simulink model "AFDNFSmodelMPA"  (Simulink 8.8)
settings: Solver=ode45  StartTime=0.0  StopTime=100  FixedStep=1e-3  RelTol=1e-6  EnableMultiTasking=on
InitFcn:
  | run('Methods/AFDSimInit')
  | load('SampleDatcomData.mat')
values from neighbouring files (symbols this model uses):
  nfs = TransferFunction('Plot','true')    [Main.m]    (also in NFSDatabase.sldd = SI
                Imperial
                28184.4409185639)
undefined symbols (not defined in the file or in its folder): datcom, desired, K_lat, K_long, Kobsvlat, Kobsvlong, lat, latsys, long, longsys, Newton, Raphson, sigbuilder_block
libraries: aerolibutil x13, aerolibtransform2 x1, aerolibasang x1
(part 3 of 3)

== system AFDNFSmodelMPA/Nonlinear Flight Simulator/Forces&Moments/Digital DATCOM v1.0.2/Deflection/Aerodynamic Forces and Moments/CG-CP Transformation/Body2Stability ==
  alpha : Inport
  Constant{,1,3..4} (4 alike) : Constant  Value=0
  Constant2 : Constant
  Create 3x3 Matrix : aerolibutil/Create 3x3 Matrix
  Trigonometric Function2 : Trigonometry  Operator=sincos
  Unary Minus : UnaryMinus
  Ts/b : Outport
  wires:
  alpha/1 -> Trigonometric Function2/1
  Trigonometric Function2/2 -> Create 3x3 Matrix/9, Create 3x3 Matrix/1
  Constant4/1 -> Create 3x3 Matrix/8
  Unary Minus/1 -> Create 3x3 Matrix/7
  Trigonometric Function2/1 -> Unary Minus/1, Create 3x3 Matrix/3
  Constant3/1 -> Create 3x3 Matrix/6
  Constant2/1 -> Create 3x3 Matrix/5
  Constant1/1 -> Create 3x3 Matrix/4
  Constant/1 -> Create 3x3 Matrix/2
  Create 3x3 Matrix/1 -> Ts/b/1

== system AFDNFSmodelMPA/Nonlinear Flight Simulator/Forces&Moments/Digital DATCOM v1.0.2/Deflection/Aerodynamic Forces and Moments/CG-CP Transformation/Incidence, Sideslip, & Airspeed ==
  Vb : Inport  Unit=m/s
  Airspeed : Sqrt  AlgorithmType=Newton-Raphson  SaturateOnIntegerOverflow=on
  Dot Product : DotProduct  InputSameDT=on  OutDataTypeStr=Inherit: Inherit via internal rule
  Incidence : Trigonometry  Operator=atan2
  Product : Product  Inputs=*/  SaturateOnIntegerOverflow=on  OutDataTypeStr=Inherit: Same as first input
  Selector : Selector  InputPortWidth=3  IndexOptions=Index vector (dialog)  Indices=[2]  OutputSizes=1
  Selector1 : Selector  InputPortWidth=3  IndexOptions=Index vector (dialog)  Indices=[3]  OutputSizes=1
  Selector2 : Selector  InputPortWidth=3  IndexOptions=Index vector (dialog)  Indices=[1]  OutputSizes=1
  Sideslip : Trigonometry  Operator=asin
  Alpha : Outport  Unit=rad  InitialOutput=0
  Beta : Outport  Port=2  Unit=rad  InitialOutput=0
  V : Outport  Port=3  Unit=m/s  InitialOutput=0
  wires:
  Selector/1 -> Product/1
  Sideslip/1 -> Beta/1
  Vb/1 -> Dot Product/2, Dot Product/1, Selector/1, Selector2/1, Selector1/1
  Incidence/1 -> Alpha/1
  Airspeed/1 -> V/1, Product/2
  Dot Product/1 -> Airspeed/1
  Selector2/1 -> Incidence/2
  Selector1/1 -> Incidence/1
  Product/1 -> Sideslip/1

== system AFDNFSmodelMPA/Nonlinear Flight Simulator/Forces&Moments/Digital DATCOM v1.0.2/Deflection/Aerodynamic Forces and Moments/Force Transformation/Body2Stability ==
  alpha : Inport
  Constant{,1,3..4} (4 alike) : Constant  Value=0
  Constant2 : Constant
  Create 3x3 Matrix : aerolibutil/Create 3x3 Matrix
  Trigonometric Function2 : Trigonometry  Operator=sincos
  Unary Minus : UnaryMinus
  Ts/b : Outport
  wires:
  alpha/1 -> Trigonometric Function2/1
  Trigonometric Function2/2 -> Create 3x3 Matrix/9, Create 3x3 Matrix/1
  Constant4/1 -> Create 3x3 Matrix/8
  Unary Minus/1 -> Create 3x3 Matrix/7
  Trigonometric Function2/1 -> Unary Minus/1, Create 3x3 Matrix/3
  Constant3/1 -> Create 3x3 Matrix/6
  Constant2/1 -> Create 3x3 Matrix/5
  Constant1/1 -> Create 3x3 Matrix/4
  Constant/1 -> Create 3x3 Matrix/2
  Create 3x3 Matrix/1 -> Ts/b/1

== system AFDNFSmodelMPA/Nonlinear Flight Simulator/Forces&Moments/Digital DATCOM v1.0.2/Deflection/Aerodynamic Forces and Moments/Force Transformation/Incidence, Sideslip, & Airspeed ==
  Vb : Inport  Unit=m/s
  Airspeed : Sqrt  AlgorithmType=Newton-Raphson  SaturateOnIntegerOverflow=on
  Dot Product : DotProduct  InputSameDT=on  OutDataTypeStr=Inherit: Inherit via internal rule
  Incidence : Trigonometry  Operator=atan2
  Product : Product  Inputs=*/  SaturateOnIntegerOverflow=on  OutDataTypeStr=Inherit: Same as first input
  Selector : Selector  InputPortWidth=3  IndexOptions=Index vector (dialog)  Indices=[2]  OutputSizes=1
  Selector1 : Selector  InputPortWidth=3  IndexOptions=Index vector (dialog)  Indices=[3]  OutputSizes=1
  Selector2 : Selector  InputPortWidth=3  IndexOptions=Index vector (dialog)  Indices=[1]  OutputSizes=1
  Sideslip : Trigonometry  Operator=asin
  Alpha : Outport  Unit=rad  InitialOutput=0
  Beta : Outport  Port=2  Unit=rad  InitialOutput=0
  V : Outport  Port=3  Unit=m/s  InitialOutput=0
  wires:
  Selector/1 -> Product/1
  Sideslip/1 -> Beta/1
  Vb/1 -> Dot Product/2, Dot Product/1, Selector/1, Selector2/1, Selector1/1
  Incidence/1 -> Alpha/1
  Airspeed/1 -> V/1, Product/2
  Dot Product/1 -> Airspeed/1
  Selector2/1 -> Incidence/2
  Selector1/1 -> Incidence/1
  Product/1 -> Sideslip/1

== system AFDNFSmodelMPA/Nonlinear Flight Simulator/Forces&Moments/Digital DATCOM v1.0.2/Deflection/Aerodynamic Forces and Moments/Moment Transformation/Body2Stability ==
  alpha : Inport
  Constant{,1,3..4} (4 alike) : Constant  Value=0
  Constant2 : Constant
  Create 3x3 Matrix : aerolibutil/Create 3x3 Matrix
  Trigonometric Function2 : Trigonometry  Operator=sincos
  Unary Minus : UnaryMinus
  Ts/b : Outport
  wires:
  Create 3x3 Matrix/1 -> Ts/b/1
  Constant/1 -> Create 3x3 Matrix/2
  Constant1/1 -> Create 3x3 Matrix/4
  Constant2/1 -> Create 3x3 Matrix/5
  Constant3/1 -> Create 3x3 Matrix/6
  Trigonometric Function2/1 -> Create 3x3 Matrix/3, Unary Minus/1
  Unary Minus/1 -> Create 3x3 Matrix/7
  Constant4/1 -> Create 3x3 Matrix/8
  Trigonometric Function2/2 -> Create 3x3 Matrix/1, Create 3x3 Matrix/9
  alpha/1 -> Trigonometric Function2/1

== system AFDNFSmodelMPA/Nonlinear Flight Simulator/Forces&Moments/Digital DATCOM v1.0.2/Deflection/Aerodynamic Forces and Moments/Moment Transformation/Incidence, Sideslip, & Airspeed ==
  Vb : Inport  Unit=m/s
  Airspeed : Sqrt  AlgorithmType=Newton-Raphson  SaturateOnIntegerOverflow=on
  Dot Product : DotProduct  InputSameDT=on  OutDataTypeStr=Inherit: Inherit via internal rule
  Incidence : Trigonometry  Operator=atan2
  Product : Product  Inputs=*/  SaturateOnIntegerOverflow=on  OutDataTypeStr=Inherit: Same as first input
  Selector : Selector  InputPortWidth=3  IndexOptions=Index vector (dialog)  Indices=[2]  OutputSizes=1
  Selector1 : Selector  InputPortWidth=3  IndexOptions=Index vector (dialog)  Indices=[3]  OutputSizes=1
  Selector2 : Selector  InputPortWidth=3  IndexOptions=Index vector (dialog)  Indices=[1]  OutputSizes=1
  Sideslip : Trigonometry  Operator=asin
  Alpha : Outport  Unit=rad  InitialOutput=0
  Beta : Outport  Port=2  Unit=rad  InitialOutput=0
  V : Outport  Port=3  Unit=m/s  InitialOutput=0
  wires:
  Product/1 -> Sideslip/1
  Selector1/1 -> Incidence/1
  Selector2/1 -> Incidence/2
  Dot Product/1 -> Airspeed/1
  Airspeed/1 -> Product/2, V/1
  Incidence/1 -> Alpha/1
  Vb/1 -> Selector1/1, Selector2/1, Selector/1, Dot Product/1, Dot Product/2
  Sideslip/1 -> Beta/1
  Selector/1 -> Product/1

== system AFDNFSmodelMPA/Nonlinear Flight Simulator/Forces&Moments/Digital DATCOM v1.0.2/Dynamic Contribution/Aerodynamic Forces and Moments Stability Axis/CG-CP Transformation/Body2Stability ==
  alpha : Inport
  Constant{,1,3..4} (4 alike) : Constant  Value=0
  Constant2 : Constant
  Create 3x3 Matrix : aerolibutil/Create 3x3 Matrix
  Trigonometric Function2 : Trigonometry  Operator=sincos
  Unary Minus : UnaryMinus
  Ts/b : Outport
  wires:
  alpha/1 -> Trigonometric Function2/1
  Trigonometric Function2/2 -> Create 3x3 Matrix/9, Create 3x3 Matrix/1
  Constant4/1 -> Create 3x3 Matrix/8
  Unary Minus/1 -> Create 3x3 Matrix/7
  Trigonometric Function2/1 -> Unary Minus/1, Create 3x3 Matrix/3
  Constant3/1 -> Create 3x3 Matrix/6
  Constant2/1 -> Create 3x3 Matrix/5
  Constant1/1 -> Create 3x3 Matrix/4
  Constant/1 -> Create 3x3 Matrix/2
  Create 3x3 Matrix/1 -> Ts/b/1

== system AFDNFSmodelMPA/Nonlinear Flight Simulator/Forces&Moments/Digital DATCOM v1.0.2/Dynamic Contribution/Aerodynamic Forces and Moments Stability Axis/CG-CP Transformation/Incidence, Sideslip, & Airspeed ==
  Vb : Inport  Unit=m/s
  Airspeed : Sqrt  AlgorithmType=Newton-Raphson  SaturateOnIntegerOverflow=on
  Dot Product : DotProduct  InputSameDT=on  OutDataTypeStr=Inherit: Inherit via internal rule
  Incidence : Trigonometry  Operator=atan2
  Product : Product  Inputs=*/  SaturateOnIntegerOverflow=on  OutDataTypeStr=Inherit: Same as first input
  Selector : Selector  InputPortWidth=3  IndexOptions=Index vector (dialog)  Indices=[2]  OutputSizes=1
  Selector1 : Selector  InputPortWidth=3  IndexOptions=Index vector (dialog)  Indices=[3]  OutputSizes=1
  Selector2 : Selector  InputPortWidth=3  IndexOptions=Index vector (dialog)  Indices=[1]  OutputSizes=1
  Sideslip : Trigonometry  Operator=asin
  Alpha : Outport  Unit=rad  InitialOutput=0
  Beta : Outport  Port=2  Unit=rad  InitialOutput=0
  V : Outport  Port=3  Unit=m/s  InitialOutput=0
  wires:
  Selector/1 -> Product/1
  Sideslip/1 -> Beta/1
  Vb/1 -> Dot Product/2, Dot Product/1, Selector/1, Selector2/1, Selector1/1
  Incidence/1 -> Alpha/1
  Airspeed/1 -> V/1, Product/2
  Dot Product/1 -> Airspeed/1
  Selector2/1 -> Incidence/2
  Selector1/1 -> Incidence/1
  Product/1 -> Sideslip/1

== system AFDNFSmodelMPA/Nonlinear Flight Simulator/Forces&Moments/Digital DATCOM v1.0.2/Dynamic Contribution/Aerodynamic Forces and Moments Stability Axis/Force Transformation/Body2Stability ==
  alpha : Inport
  Constant{,1,3..4} (4 alike) : Constant  Value=0
  Constant2 : Constant
  Create 3x3 Matrix : aerolibutil/Create 3x3 Matrix
  Trigonometric Function2 : Trigonometry  Operator=sincos
  Unary Minus : UnaryMinus
  Ts/b : Outport
  wires:
  alpha/1 -> Trigonometric Function2/1
  Trigonometric Function2/2 -> Create 3x3 Matrix/9, Create 3x3 Matrix/1
  Constant4/1 -> Create 3x3 Matrix/8
  Unary Minus/1 -> Create 3x3 Matrix/7
  Trigonometric Function2/1 -> Unary Minus/1, Create 3x3 Matrix/3
  Constant3/1 -> Create 3x3 Matrix/6
  Constant2/1 -> Create 3x3 Matrix/5
  Constant1/1 -> Create 3x3 Matrix/4
  Constant/1 -> Create 3x3 Matrix/2
  Create 3x3 Matrix/1 -> Ts/b/1

== system AFDNFSmodelMPA/Nonlinear Flight Simulator/Forces&Moments/Digital DATCOM v1.0.2/Dynamic Contribution/Aerodynamic Forces and Moments Stability Axis/Force Transformation/Incidence, Sideslip, & Airspeed ==
  Vb : Inport  Unit=m/s
  Airspeed : Sqrt  AlgorithmType=Newton-Raphson  SaturateOnIntegerOverflow=on
  Dot Product : DotProduct  InputSameDT=on  OutDataTypeStr=Inherit: Inherit via internal rule
  Incidence : Trigonometry  Operator=atan2
  Product : Product  Inputs=*/  SaturateOnIntegerOverflow=on  OutDataTypeStr=Inherit: Same as first input
  Selector : Selector  InputPortWidth=3  IndexOptions=Index vector (dialog)  Indices=[2]  OutputSizes=1
  Selector1 : Selector  InputPortWidth=3  IndexOptions=Index vector (dialog)  Indices=[3]  OutputSizes=1
  Selector2 : Selector  InputPortWidth=3  IndexOptions=Index vector (dialog)  Indices=[1]  OutputSizes=1
  Sideslip : Trigonometry  Operator=asin
  Alpha : Outport  Unit=rad  InitialOutput=0
  Beta : Outport  Port=2  Unit=rad  InitialOutput=0
  V : Outport  Port=3  Unit=m/s  InitialOutput=0
  wires:
  Selector/1 -> Product/1
  Sideslip/1 -> Beta/1
  Vb/1 -> Dot Product/2, Dot Product/1, Selector/1, Selector2/1, Selector1/1
  Incidence/1 -> Alpha/1
  Airspeed/1 -> V/1, Product/2
  Dot Product/1 -> Airspeed/1
  Selector2/1 -> Incidence/2
  Selector1/1 -> Incidence/1
  Product/1 -> Sideslip/1

== system AFDNFSmodelMPA/Nonlinear Flight Simulator/Forces&Moments/Digital DATCOM v1.0.2/Dynamic Contribution/Aerodynamic Forces and Moments Stability Axis/Moment Transformation/Body2Stability ==
  alpha : Inport
  Constant{,1,3..4} (4 alike) : Constant  Value=0
  Constant2 : Constant
  Create 3x3 Matrix : aerolibutil/Create 3x3 Matrix
  Trigonometric Function2 : Trigonometry  Operator=sincos
  Unary Minus : UnaryMinus
  Ts/b : Outport
  wires:
  Create 3x3 Matrix/1 -> Ts/b/1
  Constant/1 -> Create 3x3 Matrix/2
  Constant1/1 -> Create 3x3 Matrix/4
  Constant2/1 -> Create 3x3 Matrix/5
  Constant3/1 -> Create 3x3 Matrix/6
  Trigonometric Function2/1 -> Create 3x3 Matrix/3, Unary Minus/1
  Unary Minus/1 -> Create 3x3 Matrix/7
  Constant4/1 -> Create 3x3 Matrix/8
  Trigonometric Function2/2 -> Create 3x3 Matrix/1, Create 3x3 Matrix/9
  alpha/1 -> Trigonometric Function2/1

== system AFDNFSmodelMPA/Nonlinear Flight Simulator/Forces&Moments/Digital DATCOM v1.0.2/Dynamic Contribution/Aerodynamic Forces and Moments Stability Axis/Moment Transformation/Incidence, Sideslip, & Airspeed ==
  Vb : Inport  Unit=m/s
  Airspeed : Sqrt  AlgorithmType=Newton-Raphson  SaturateOnIntegerOverflow=on
  Dot Product : DotProduct  InputSameDT=on  OutDataTypeStr=Inherit: Inherit via internal rule
  Incidence : Trigonometry  Operator=atan2
  Product : Product  Inputs=*/  SaturateOnIntegerOverflow=on  OutDataTypeStr=Inherit: Same as first input
  Selector : Selector  InputPortWidth=3  IndexOptions=Index vector (dialog)  Indices=[2]  OutputSizes=1
  Selector1 : Selector  InputPortWidth=3  IndexOptions=Index vector (dialog)  Indices=[3]  OutputSizes=1
  Selector2 : Selector  InputPortWidth=3  IndexOptions=Index vector (dialog)  Indices=[1]  OutputSizes=1
  Sideslip : Trigonometry  Operator=asin
  Alpha : Outport  Unit=rad  InitialOutput=0
  Beta : Outport  Port=2  Unit=rad  InitialOutput=0
  V : Outport  Port=3  Unit=m/s  InitialOutput=0
  wires:
  Product/1 -> Sideslip/1
  Selector1/1 -> Incidence/1
  Selector2/1 -> Incidence/2
  Dot Product/1 -> Airspeed/1
  Airspeed/1 -> Product/2, V/1
  Incidence/1 -> Alpha/1
  Vb/1 -> Selector1/1, Selector2/1, Selector/1, Dot Product/1, Dot Product/2
  Sideslip/1 -> Beta/1
  Selector/1 -> Product/1

== system AFDNFSmodelMPA/Nonlinear Flight Simulator/Forces&Moments/Digital DATCOM v1.0.2/Static Contribution/Aerodynamic Forces and Moments/CG-CP Transformation/Body2Stability ==
  alpha : Inport
  Constant{,1,3..4} (4 alike) : Constant  Value=0
  Constant2 : Constant
  Create 3x3 Matrix : aerolibutil/Create 3x3 Matrix
  Trigonometric Function2 : Trigonometry  Operator=sincos
  Unary Minus : UnaryMinus
  Ts/b : Outport
  wires:
  alpha/1 -> Trigonometric Function2/1
  Trigonometric Function2/2 -> Create 3x3 Matrix/9, Create 3x3 Matrix/1
  Constant4/1 -> Create 3x3 Matrix/8
  Unary Minus/1 -> Create 3x3 Matrix/7
  Trigonometric Function2/1 -> Unary Minus/1, Create 3x3 Matrix/3
  Constant3/1 -> Create 3x3 Matrix/6
  Constant2/1 -> Create 3x3 Matrix/5
  Constant1/1 -> Create 3x3 Matrix/4
  Constant/1 -> Create 3x3 Matrix/2
  Create 3x3 Matrix/1 -> Ts/b/1

== system AFDNFSmodelMPA/Nonlinear Flight Simulator/Forces&Moments/Digital DATCOM v1.0.2/Static Contribution/Aerodynamic Forces and Moments/CG-CP Transformation/Incidence, Sideslip, & Airspeed ==
  Vb : Inport  Unit=m/s
  Airspeed : Sqrt  AlgorithmType=Newton-Raphson  SaturateOnIntegerOverflow=on
  Dot Product : DotProduct  InputSameDT=on  OutDataTypeStr=Inherit: Inherit via internal rule
  Incidence : Trigonometry  Operator=atan2
  Product : Product  Inputs=*/  SaturateOnIntegerOverflow=on  OutDataTypeStr=Inherit: Same as first input
  Selector : Selector  InputPortWidth=3  IndexOptions=Index vector (dialog)  Indices=[2]  OutputSizes=1
  Selector1 : Selector  InputPortWidth=3  IndexOptions=Index vector (dialog)  Indices=[3]  OutputSizes=1
  Selector2 : Selector  InputPortWidth=3  IndexOptions=Index vector (dialog)  Indices=[1]  OutputSizes=1
  Sideslip : Trigonometry  Operator=asin
  Alpha : Outport  Unit=rad  InitialOutput=0
  Beta : Outport  Port=2  Unit=rad  InitialOutput=0
  V : Outport  Port=3  Unit=m/s  InitialOutput=0
  wires:
  Selector/1 -> Product/1
  Sideslip/1 -> Beta/1
  Vb/1 -> Dot Product/2, Dot Product/1, Selector/1, Selector2/1, Selector1/1
  Incidence/1 -> Alpha/1
  Airspeed/1 -> V/1, Product/2
  Dot Product/1 -> Airspeed/1
  Selector2/1 -> Incidence/2
  Selector1/1 -> Incidence/1
  Product/1 -> Sideslip/1

== system AFDNFSmodelMPA/Nonlinear Flight Simulator/Forces&Moments/Digital DATCOM v1.0.2/Static Contribution/Aerodynamic Forces and Moments/Force Transformation/Body2Stability ==
  alpha : Inport
  Constant{,1,3..4} (4 alike) : Constant  Value=0
  Constant2 : Constant
  Create 3x3 Matrix : aerolibutil/Create 3x3 Matrix
  Trigonometric Function2 : Trigonometry  Operator=sincos
  Unary Minus : UnaryMinus
  Ts/b : Outport
  wires:
  alpha/1 -> Trigonometric Function2/1
  Trigonometric Function2/2 -> Create 3x3 Matrix/9, Create 3x3 Matrix/1
  Constant4/1 -> Create 3x3 Matrix/8
  Unary Minus/1 -> Create 3x3 Matrix/7
  Trigonometric Function2/1 -> Unary Minus/1, Create 3x3 Matrix/3
  Constant3/1 -> Create 3x3 Matrix/6
  Constant2/1 -> Create 3x3 Matrix/5
  Constant1/1 -> Create 3x3 Matrix/4
  Constant/1 -> Create 3x3 Matrix/2
  Create 3x3 Matrix/1 -> Ts/b/1

== system AFDNFSmodelMPA/Nonlinear Flight Simulator/Forces&Moments/Digital DATCOM v1.0.2/Static Contribution/Aerodynamic Forces and Moments/Force Transformation/Incidence, Sideslip, & Airspeed ==
  Vb : Inport  Unit=m/s
  Airspeed : Sqrt  AlgorithmType=Newton-Raphson  SaturateOnIntegerOverflow=on
  Dot Product : DotProduct  InputSameDT=on  OutDataTypeStr=Inherit: Inherit via internal rule
  Incidence : Trigonometry  Operator=atan2
  Product : Product  Inputs=*/  SaturateOnIntegerOverflow=on  OutDataTypeStr=Inherit: Same as first input
  Selector : Selector  InputPortWidth=3  IndexOptions=Index vector (dialog)  Indices=[2]  OutputSizes=1
  Selector1 : Selector  InputPortWidth=3  IndexOptions=Index vector (dialog)  Indices=[3]  OutputSizes=1
  Selector2 : Selector  InputPortWidth=3  IndexOptions=Index vector (dialog)  Indices=[1]  OutputSizes=1
  Sideslip : Trigonometry  Operator=asin
  Alpha : Outport  Unit=rad  InitialOutput=0
  Beta : Outport  Port=2  Unit=rad  InitialOutput=0
  V : Outport  Port=3  Unit=m/s  InitialOutput=0
  wires:
  Selector/1 -> Product/1
  Sideslip/1 -> Beta/1
  Vb/1 -> Dot Product/2, Dot Product/1, Selector/1, Selector2/1, Selector1/1
  Incidence/1 -> Alpha/1
  Airspeed/1 -> V/1, Product/2
  Dot Product/1 -> Airspeed/1
  Selector2/1 -> Incidence/2
  Selector1/1 -> Incidence/1
  Product/1 -> Sideslip/1

== system AFDNFSmodelMPA/Nonlinear Flight Simulator/Forces&Moments/Digital DATCOM v1.0.2/Static Contribution/Aerodynamic Forces and Moments/Moment Transformation/Body2Stability ==
  alpha : Inport
  Constant{,1,3..4} (4 alike) : Constant  Value=0
  Constant2 : Constant
  Create 3x3 Matrix : aerolibutil/Create 3x3 Matrix
  Trigonometric Function2 : Trigonometry  Operator=sincos
  Unary Minus : UnaryMinus
  Ts/b : Outport
  wires:
  Create 3x3 Matrix/1 -> Ts/b/1
  Constant/1 -> Create 3x3 Matrix/2
  Constant1/1 -> Create 3x3 Matrix/4
  Constant2/1 -> Create 3x3 Matrix/5
  Constant3/1 -> Create 3x3 Matrix/6
  Trigonometric Function2/1 -> Create 3x3 Matrix/3, Unary Minus/1
  Unary Minus/1 -> Create 3x3 Matrix/7
  Constant4/1 -> Create 3x3 Matrix/8
  Trigonometric Function2/2 -> Create 3x3 Matrix/1, Create 3x3 Matrix/9
  alpha/1 -> Trigonometric Function2/1

== system AFDNFSmodelMPA/Nonlinear Flight Simulator/Forces&Moments/Digital DATCOM v1.0.2/Static Contribution/Aerodynamic Forces and Moments/Moment Transformation/Incidence, Sideslip, & Airspeed ==
  Vb : Inport  Unit=m/s
  Airspeed : Sqrt  AlgorithmType=Newton-Raphson  SaturateOnIntegerOverflow=on
  Dot Product : DotProduct  InputSameDT=on  OutDataTypeStr=Inherit: Inherit via internal rule
  Incidence : Trigonometry  Operator=atan2
  Product : Product  Inputs=*/  SaturateOnIntegerOverflow=on  OutDataTypeStr=Inherit: Same as first input
  Selector : Selector  InputPortWidth=3  IndexOptions=Index vector (dialog)  Indices=[2]  OutputSizes=1
  Selector1 : Selector  InputPortWidth=3  IndexOptions=Index vector (dialog)  Indices=[3]  OutputSizes=1
  Selector2 : Selector  InputPortWidth=3  IndexOptions=Index vector (dialog)  Indices=[1]  OutputSizes=1
  Sideslip : Trigonometry  Operator=asin
  Alpha : Outport  Unit=rad  InitialOutput=0
  Beta : Outport  Port=2  Unit=rad  InitialOutput=0
  V : Outport  Port=3  Unit=m/s  InitialOutput=0
  wires:
  Product/1 -> Sideslip/1
  Selector1/1 -> Incidence/1
  Selector2/1 -> Incidence/2
  Dot Product/1 -> Airspeed/1
  Airspeed/1 -> Product/2, V/1
  Incidence/1 -> Alpha/1
  Vb/1 -> Selector1/1, Selector2/1, Selector/1, Dot Product/1, Dot Product/2
  Sideslip/1 -> Beta/1
  Selector/1 -> Product/1
